simulink model "MBD_W1_P8"  (R2020a)
settings: Solver=VariableStepAuto  StartTime=0.0  StopTime=10.0  RelTol=1e-3
settings Model: Creator=Atri Mondal  LastModifiedBy=Atri Mondal

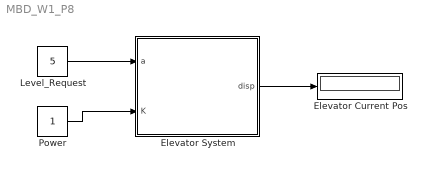
== system MBD_W1_P8 ==
  Elevator Current Pos : Display
  Elevator System : Stateflow chart  TreatAsAtomicUnit=on
  Level_Request : Constant  Value=5
  Power : Constant
  wires:
  Elevator System/1(disp) -> Elevator Current Pos/1
  Level_Request/1 -> Elevator System/1(a)
  Power/1 -> Elevator System/2(K)

== stateflow chart MBD_W1_P8/Elevator System ==
  data: a input; disp output; power local; K input
  events: inc local FUNCTION_CALL_EVENT
